simulink model "MHE"  (R2021b)
settings: Solver=FixedStepAuto  StartTime=0.0  StopTime=200  FixedStep=1e-4  RelTol=1e-3
InitFcn:
  | N = 10;
libraries: commchan3 x1
settings Model: Creator=12406  LastModifiedBy=aryal
settings SolverCC: AlgebraicLoopSolver=TrustRegion
settings DebuggingCC: ArithmeticOperatorsInVariantConditions=warning
settings SFSimCC: CustomCodeUndefinedFunction=UseInterfaceOnly

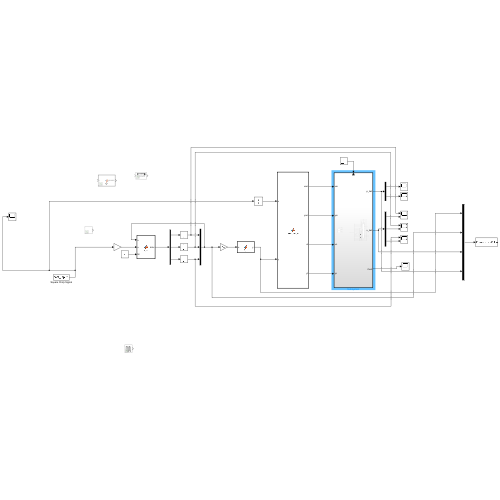
[thumbnail: Simulink's stored preview of the top-level diagram]
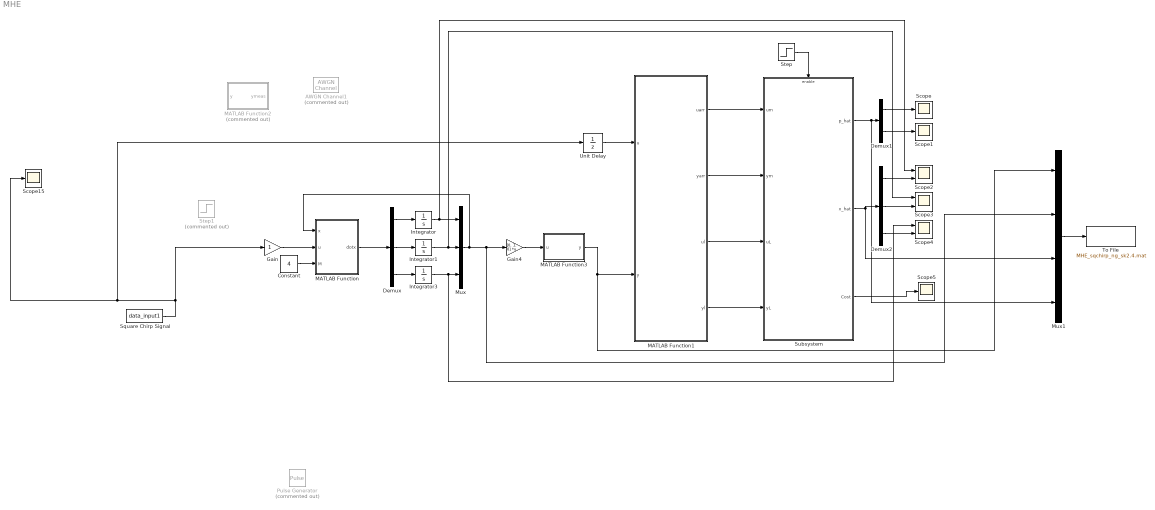
== system MHE ==
  AWGN Channel1 : commchan3/AWGN Channel  Commented=on  InputProcessing=Columns as channels (frame based)  seed=65  noiseMode=Variance from mask  EbNodB=10  EsNodB=10  SNRdB=65  bitsPerSym=1  Ps=1  Tsym=1  variance=1e-6
  Constant : Constant  Value=4
  Demux : Demux  Outputs=3
  Demux1 : Demux  Outputs=2
  Demux2 : Demux  Outputs=3
  Gain : Gain
  Gain4 : Gain  Gain=[0, 1, 0]  Multiplication=Matrix(K*u)
  Integrator : Integrator
  Integrator1 : Integrator
  Integrator3 : Integrator
  MATLAB Function : MATLAB Function  TreatAsAtomicUnit=on
  MATLAB Function1 : MATLAB Function  TreatAsAtomicUnit=on  SystemSampleTime=0.02
  MATLAB Function2 : MATLAB Function  Commented=on  TreatAsAtomicUnit=on
  MATLAB Function3 : MATLAB Function  TreatAsAtomicUnit=on
  Mux : Mux  Inputs=3
  Mux1 : Mux
  Pulse Generator : DiscretePulseGenerator  Commented=on  PulseType=Time based  Amplitude=0.2  PulseWidth=50
  Scope{,1,5,15} (4 alike) : Scope
  Scope2 : Scope  NumInputPorts=2
  Scope3 : Scope  NumInputPorts=2
  Scope4 : Scope  NumInputPorts=2
  Square Chirp Signal : FromWorkspace  VariableName=data_input1  SampleTime=0.02
  Step : Step  SampleTime=0
  Step1 : Step  Commented=on  Time=100  Before=4.0  After=6.0  SampleTime=0
  Subsystem : Subsystem
  To File : ToFile  Filename=MHE_sqchirp_ng_sk2.4.mat  MatrixName=w  SampleTime=0.02
  Unit Delay : UnitDelay  SampleTime=0.02  HasFrameUpgradeWarning=on
  wires:
  Integrator/1 -> Scope2/1, Mux/1
  Integrator1/1 -> Scope3/1, Mux/2
  Demux/3 -> Integrator3/1
  MATLAB Function/1(dotx) -> Demux/1
  Demux/2 -> Integrator1/1
  Integrator3/1 -> Scope4/1, Mux/3
  Demux/1 -> Integrator/1
  Mux/1 -> MATLAB Function/1(x), Mux1/2, Gain4/1
  Unit Delay/1 -> MATLAB Function1/1(u)
  Subsystem/1(p_hat) -> Mux1/4, Demux1/1
  Demux1/1 -> Scope/1
  Demux1/2 -> Scope1/1
  Mux1/1 -> To File/1
  Gain/1 -> MATLAB Function/2(u)
  Square Chirp Signal/1 -> Gain/1, Unit Delay/1, Scope15/1
  Step/1 -> Subsystem/Enable
  Subsystem/2(x_hat) -> Demux2/1, Mux1/3
  Demux2/1 -> Scope2/2
  Demux2/2 -> Scope3/2
  Demux2/3 -> Scope4/2
  Constant/1 -> MATLAB Function/3(M)
  Gain4/1 -> MATLAB Function3/1(u)
  Subsystem/3(Cost) -> Scope5/1
  MATLAB Function1/1(uarr) -> Subsystem/1(um)
  MATLAB Function1/2(yarr) -> Subsystem/2(ym)
  MATLAB Function1/4(yl) -> Subsystem/4(yL)
  MATLAB Function1/3(ul) -> Subsystem/3(uL)
  MATLAB Function3/1(y) -> Mux1/1, MATLAB Function1/2(y)

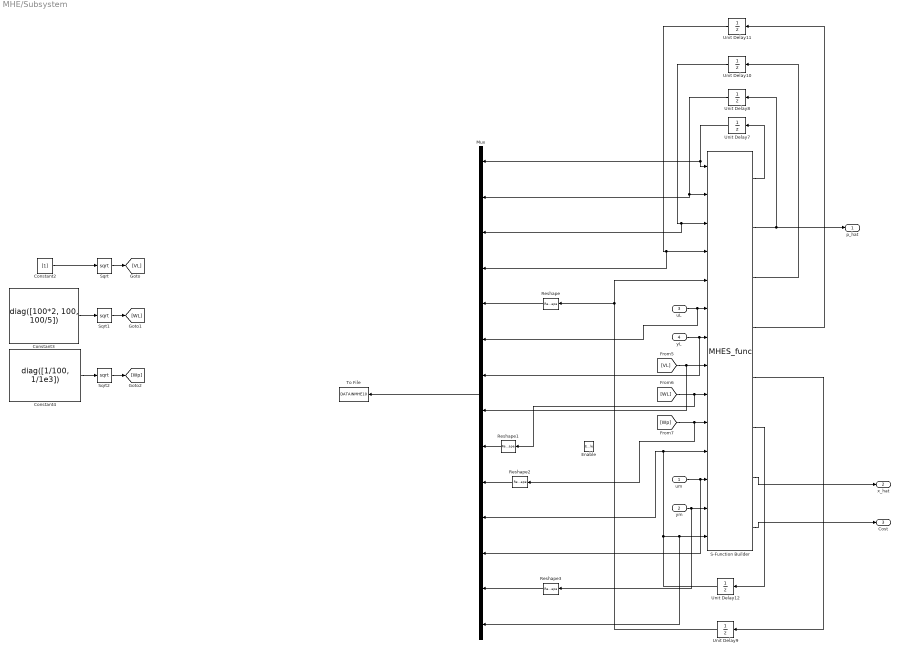
== system MHE/Subsystem ==
  um : Inport
  ym : Inport  Port=2
  uL : Inport  Port=3
  yL : Inport  Port=4
  Enable : EnablePort
  Constant2 : Constant  Value=[1]
  Constant3 : Constant  Value=diag([100*2, 100, 100/5])
  Constant4 : Constant  Value=diag([1/100, 1/1e3])
  Mux : Mux  Inputs=14
  Reshape{,1..3} (4 alike) : Reshape
  S-Function Builder : S-Function  FunctionName=MHES_func  SFunctionModules=MHES_func_wrapper MHEArrival MHEArrival_Call  SFunctionDeploymentMode=off  EnableBusSupport=off  mask(S-Function Builder){}
      mask help: Simulink:masks:SFunctionBuilder_MD
      mask init:
      | val = [[.9  0.75 0.75 1 1 .9 .9 1]',[1 1 0.75 0.75 .9 .9 1 .9]'];try , sys = get_param(gcb,'SfunBuilderFcnName');if isempty(sys), sys = get_param(gcb,'FunctionName'); end,catch, sys = get_param(gcb,'FunctionName'); end
      settings: CopyFcn=set_param(gcbh,'LinkStatus','none')  OpenFcn=sfunctionwizard(gcbh)
      mask Display:
      | plot(val(:,1),val(:,2))
      | disp(sys)
      | port_label('input',1,'xL')
      | port_label('input',2,'pL')
      | port_label('input',3,'xLb')
      | port_label('input',4,'pLb')
      | port_label('input',5,'PL')
      | port_label('input',6,'uL')
      | port_label('input',7,'yL')
      | port_label('input',8,'VL')
      | port_label('input',9,'WL')
      | port_label('input',10,'Wp')
      | port_label('input',11,'zGuess')
      | port_label('input',12,'um')
      | port_label('input',13,'ym')
      | port_label('input',14,'zOp')
      | port_label('output',1,'xLout')
      | port_label('output',2,'p_hat')
      | port_label('output',3,'xLbn')
      | port_label('output',4,'pLbn')
      | port_label('output',5,'PLn')
      | port_label('output',6,'zOut')
      | port_label('output',7,'x_hat')
      | port_label('output',8,'Cost')
  Sqrt : Sqrt  SaturateOnIntegerOverflow=on
  Sqrt1 : Sqrt  SaturateOnIntegerOverflow=on
  Sqrt2 : Sqrt  SaturateOnIntegerOverflow=on
  To File : ToFile  Filename=DATAINMHE10  MatrixName=W  SampleTime=0.02
  Unit Delay10 : UnitDelay  InitialCondition=zeros(3, 1)  SampleTime=0.02  HasFrameUpgradeWarning=on
  Unit Delay11 : UnitDelay  InitialCondition=[0.05, 0.05]  SampleTime=0.02  HasFrameUpgradeWarning=on
  Unit Delay12 : UnitDelay  InitialCondition=[0.05; 0.05; zeros(3*(N+1), 1)]  SampleTime=0.02  HasFrameUpgradeWarning=on
  Unit Delay7 : UnitDelay  InitialCondition=zeros(3, 1)  SampleTime=0.02  HasFrameUpgradeWarning=on
  Unit Delay8 : UnitDelay  InitialCondition=[0.05, 0.05]  SampleTime=0.02  HasFrameUpgradeWarning=on
  Unit Delay9 : UnitDelay  SampleTime=0.02  HasFrameUpgradeWarning=on
  p_hat : Outport
  x_hat : Outport  Port=2
  Cost : Outport  Port=3
  wires:
  Sqrt/1 -> [VL]
  Constant2/1 -> Sqrt/1
  Sqrt1/1 -> [WL]
  Constant3/1 -> Sqrt1/1
  Sqrt2/1 -> [Wp]
  Constant4/1 -> Sqrt2/1
  S-Function Builder/1 -> Unit Delay7/1
  Unit Delay7/1 -> Mux/1, S-Function Builder/1
  S-Function Builder/2 -> p_hat/1, Unit Delay8/1
  Unit Delay8/1 -> Mux/2, S-Function Builder/2
  S-Function Builder/3 -> Unit Delay10/1
  S-Function Builder/4 -> Unit Delay11/1
  Unit Delay11/1 -> Mux/4, S-Function Builder/4
  S-Function Builder/5 -> Unit Delay9/1
  S-Function Builder/6 -> Unit Delay12/1
  Unit Delay12/1 -> Mux/14, S-Function Builder/14, S-Function Builder/11, Mux/11
  Unit Delay9/1 -> Reshape/1, S-Function Builder/5
  uL/1 -> Mux/6, S-Function Builder/6
  [VL] -> Mux/8, S-Function Builder/8
  [WL] -> Reshape1/1, S-Function Builder/9
  [Wp] -> Reshape2/1, S-Function Builder/10
  S-Function Builder/7 -> x_hat/1
  S-Function Builder/8 -> Cost/1
  yL/1 -> S-Function Builder/7, Mux/7
  um/1 -> Mux/12, S-Function Builder/12
  ym/1 -> Reshape3/1, S-Function Builder/13
  Unit Delay10/1 -> Mux/3, S-Function Builder/3
  Mux/1 -> To File/1
  Reshape/1 -> Mux/5
  Reshape1/1 -> Mux/9
  Reshape2/1 -> Mux/10
  Reshape3/1 -> Mux/13

== matlab function MHE/MATLAB Function1 ==
  data: u input; uarr output; y input; yarr output; ul output; yl output
function [uarr, yarr, ul, yl] = DataCollect(u, y)
    N=10;

    nu=1;
    ny=1;

    persistent yData uData;
    if isempty(uData)
        yData = zeros(ny, N+1);
        uData = zeros(nu, N);
    end

    ul = uData(:, 1);
    yl = yData(:, 1);

    for k=1:N
        yData(:,k) = yData(:,k+1);
    end

    for k=1:N-1
        uData(:,k) = uData(:,k+1);
    end

    yData(:,N+1) = y;
    uData(:, N) = u;

    uarr = uData;
    yarr = yData;
end

== matlab function MHE/MATLAB Function ==
  data: x input; u input; dotx output; M input
function dotx  = fcn(x, u, M)
    D = 1.5;
%     M = 4.0;
    Tg = 0.2;
    Rp = 0.05;
    Ki=2;
   dotx=zeros(3,1);
    x1 = x(1);
    x2 = x(2);
    x3 = x(3);
    dotx = [x2;x3;-Ki/(M*Tg)*x1-(D/(M*Tg)+1/(Rp*M*Tg))*x2-(D/M+1/Tg)*x3-1/(M*Tg)*u];

== matlab function MHE/MATLAB Function2 ==
  settings: updateMethod=DISCRETE
  data: y input; ymeas output
function ymeas = fcn(y)
    coder.extrinsic('gmdistribution');
    persistent gm;
    if isempty(gm)
        mu=[-0.1832;0.1601;-0.2891];
        sigma=cat(3,[0.0767],[0.0071],[0.0557]);
        w=[0.4719,0.3184,0.2097];
        gm=gmdistribution(mu,sigma,w);
    end
    noise = 0.0;
    noise = random(gm, 1);
    ymeas = y + 5e-3/0.2884*noise;
end

== matlab function MHE/MATLAB Function3 ==
  settings: updateMethod=DISCRETE
  data: u input; y output
function y = fcn(u)

y = pearsrnd(0,1e-3,2.4,7)+u;
